simulink model "uz_pmsm_model_6LUT_pd"  (R2023b)
settings: Solver=FixedStepAuto  StartTime=0.0  StopTime=0.05  RelTol=1e-3
PreLoadFcn:
  | uz_pmsm_model_init_parameter
PostLoadFcn:
  | % Import the data from Excel for a lookup table
  | FluxMapData = readtable('C:\Users\Philipp\ultrazohm\ultrazohm_sw\ip_cores\uz_pmsm_model\FluxMapData_2023-05-26_13-07-57.csv');
  | % Row indices for lookup table
  | d_current_in_d_axis = FluxMapData(8:27,1:end);
  | % Column indices for lookup table
  | q_current_in_d_axis = FluxMapData(29:48,1:end);
  | % Output values for lookup table
  | d_Flux_d_axis = FluxMapData(50:69,1:end);
values from neighbouring files (symbols this model uses):
  ad1 = 7.2940    (= 7.294)    [LUT_approx_methode1_u_2b.m]    (also in LUT_approx_methode1_u_2b_alt.m; LUT_approx_methode2a.m = ad_1(1); LUT_approx_methode_2a_FEM.m = ad_1(1); LUT_approx_new.m = ad_1(1))
  ad2 = 0.0001    [LUT_approx_methode1_u_2b.m]    (also in LUT_approx_methode1_u_2b_alt.m; LUT_approx_methode2a.m = ad_1(2); LUT_approx_methode_2a_FEM.m = ad_1(2); LUT_approx_new.m = ad_1(2))
  ad3 = -15.5992    [LUT_approx_methode1_u_2b.m]    (also in LUT_approx_methode1_u_2b_alt.m; LUT_approx_methode2a.m = ad_1(3); LUT_approx_methode_2a_FEM.m = ad_1(3); LUT_approx_new.m = ad_1(3))
  ad4 = -186.4725    [LUT_approx_methode1_u_2b.m]    (also in LUT_approx_methode1_u_2b_alt.m; LUT_approx_methode2a.m = ad_3_6(1); LUT_approx_methode_2a_FEM.m = ad_3_6(1); LUT_approx_new.m = ad_3_6(1))
  ad5 = 187.4853    [LUT_approx_methode1_u_2b.m]    (also in LUT_approx_methode1_u_2b_alt.m; LUT_approx_methode2a.m = ad_3_6(2); LUT_approx_methode_2a_FEM.m = ad_3_6(2); LUT_approx_new.m = ad_3_6(2))
  ad6 = 0.0000    (= 0)    [LUT_approx_methode1_u_2b.m]    (also in LUT_approx_methode1_u_2b_alt.m; LUT_approx_methode2a.m = ad_3_6(3); LUT_approx_methode_2a_FEM.m = ad_3_6(3); LUT_approx_new.m = ad_3_6(3))
  aq1 = 0.0041    [LUT_approx_methode1_u_2b.m]    (also in LUT_approx_methode1_u_2b_alt.m; LUT_approx_methode2a.m = aq_1(1); LUT_approx_methode_2a_FEM.m = aq_1(1); LUT_approx_new.m = aq_1(1))
  aq2 = 0.2092    [LUT_approx_methode1_u_2b.m]    (also in LUT_approx_methode1_u_2b_alt.m; LUT_approx_methode2a.m = aq_1(2); LUT_approx_methode_2a_FEM.m = aq_1(2); LUT_approx_new.m = aq_1(2))
  aq3 = 0.0010    (= 0.001)    [LUT_approx_methode1_u_2b.m]    (also in LUT_approx_methode1_u_2b_alt.m; LUT_approx_methode2a.m = aq_1(3); LUT_approx_methode_2a_FEM.m = aq_1(3); LUT_approx_new.m = aq_1(3))
  aq4 = 28.4940    (= 28.494)    [LUT_approx_methode1_u_2b.m]    (also in LUT_approx_methode1_u_2b_alt.m; LUT_approx_methode2a.m = aq_3_6(1); LUT_approx_methode_2a_FEM.m = aq_3_6(1); LUT_approx_new.m = aq_3_6(1))
  aq5 = -24.2348    [LUT_approx_methode1_u_2b.m]    (also in LUT_approx_methode1_u_2b_alt.m; LUT_approx_methode2a.m = aq_3_6(2); LUT_approx_methode_2a_FEM.m = aq_3_6(2); LUT_approx_new.m = aq_3_6(2))
  aq6 = 0.0405    [LUT_approx_methode1_u_2b.m]    (also in LUT_approx_methode1_u_2b_alt.m; LUT_approx_methode2a.m = aq_3_6(3); LUT_approx_methode_2a_FEM.m = aq_3_6(3); LUT_approx_new.m = aq_3_6(3))
  d_current_d_Flux = FluxMapData{1,1:20}    [uz_pmsm_model_6LUT_pd_init_parameter.m]
  d_current_q_Flux = FluxMapData{66,1:20}    [uz_pmsm_model_6LUT_pd_init_parameter.m]
  entkopplung_dynamic = false    [uz_pmsm_model_6LUT_pd_init_parameter.m]
  entkopplung_linear = true    [uz_pmsm_model_6LUT_pd_init_parameter.m]
  entkopplung_static = false    [uz_pmsm_model_6LUT_pd_init_parameter.m]
  Fid1_Giq1 = ((1/2).*(aq3-aq6).*((q_current_set).^2))+((aq1./aq2).*log(cosh(aq2.*q_current_set)))-((aq4/aq5).*log(cosh(aq5.*q_current_set)))    [LUT_approx_methode2a.m]    (also in LUT_approx_methode_2a_FEM.m = (1/2).*(aq3-aq6).*((q_current_set).^2)+((aq1./aq2).*log(cosh; LUT_approx_new.m = (1/2)*(aq3-aq6)*((q_current_set).^2)+((aq1/aq2)*log(cosh(aq2; LUT_approximation_fitting.m = (1/2)*(aq3-aq6)*((iq1)^2)+((aq1/aq2)*log(cosh(aq2*iq1)))-((a)
  Fid2_Giq2 = ((ad1./ad2).*(log(cosh(ad2.*(d_current_set-ad3))))) - ((ad4./ad5).*(log(cosh(ad5.*(d_current_set-ad6)))))    [LUT_approx_methode2a.m]    (also in LUT_approx_methode_2a_FEM.m = ((ad1./ad2).*(log(cosh(ad2.*(d_current_set-ad3))))) - (((ad1)
  Flux_d = FluxMapData{43:62,1:20}'*(1e-3)    [uz_pmsm_model_6LUT_pd_init_parameter.m]
  Flux_q = FluxMapData{108:127,1:20}'*(1e-3)    [uz_pmsm_model_6LUT_pd_init_parameter.m]
  friction_coefficient = 0.001    [uz_pmsm_model_6LUT_pd_init_parameter.m]
  inertia = 0.000084    (= 8.4e-05)    [uz_pmsm_model_6LUT_pd_init_parameter.m]
  L_d = 0.00045    [uz_pmsm_model_6LUT_pd_init_parameter.m]
  L_q = 0.002    [uz_pmsm_model_6LUT_pd_init_parameter.m]
  parameter_nachfuerung = true    [uz_pmsm_model_6LUT_pd_init_parameter.m]
  polepair = 4    [uz_pmsm_model_6LUT_pd_init_parameter.m]
  praediktion_entkopplung_nonlinear = true    [uz_pmsm_model_6LUT_pd_init_parameter.m]
  psi_pm = 0.0194    [uz_pmsm_model_6LUT_pd_init_parameter.m]
  q_current_d_Flux = FluxMapData{22:41,1}    [uz_pmsm_model_6LUT_pd_init_parameter.m]
  q_current_q_Flux = FluxMapData{87:106,1}    [uz_pmsm_model_6LUT_pd_init_parameter.m]
  R_1 = 0.3    [uz_pmsm_model_6LUT_pd_init_parameter.m]
  simulate_mechanical = false    [uz_pmsm_model_6LUT_pd_init_parameter.m]
  simulate_nonlinear_modell = true    [uz_pmsm_model_6LUT_pd_init_parameter.m]
  simulate_open_loop = false    [uz_pmsm_model_6LUT_pd_init_parameter.m]
  static_friction_torque = 0.01    [uz_pmsm_model_6LUT_pd_init_parameter.m]
  tau_sum = 2*ts_regler    (= 8e-05)    [uz_pmsm_model_6LUT_pd_init_parameter.m]
  ts = 1/5e5    (= 2e-06)    [uz_pmsm_model_6LUT_pd_init_parameter.m]
  ts_regler = 1/25e3    (= 4e-05)    [uz_pmsm_model_6LUT_pd_init_parameter.m]
undefined symbols (not defined in the file or in its folder): Ki_Bo_d, Ki_Bo_q, Kp_Bo_d, Kp_Bo_q, Ldq
libraries: slpidlib x2
(part 2 of 2)

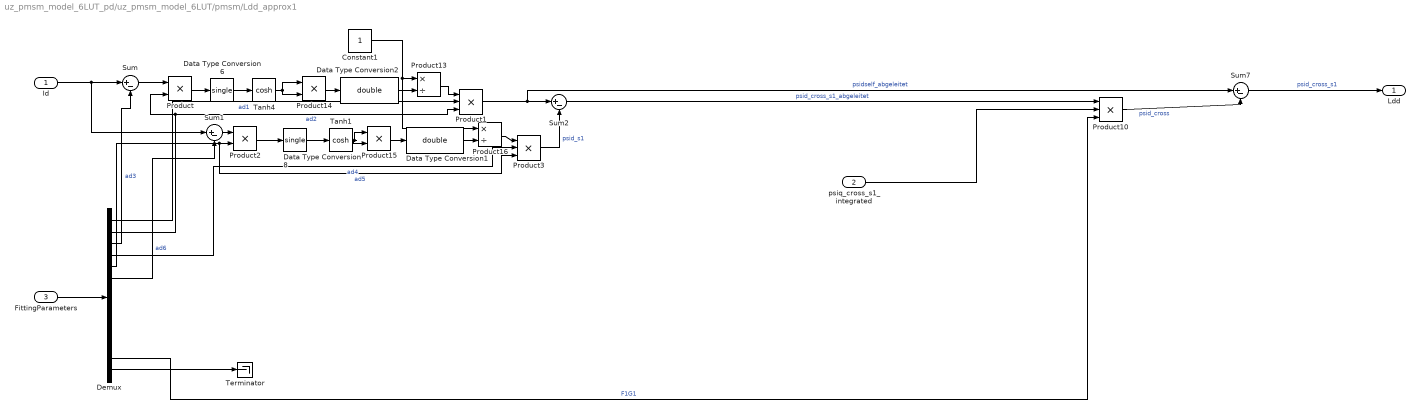
== system uz_pmsm_model_6LUT_pd/uz_pmsm_model_6LUT/pmsm/Ldd_approx1 ==
  Id : Inport
  psiq_cross_s1_integrated : Inport  Port=2
  FittingParameters : Inport  Port=3
  Constant1 : Constant  SampleTime=ts
  Data Type Conversion1 : DataTypeConversion  OutDataTypeStr=double  RndMeth=Nearest  SaturateOnIntegerOverflow=off
  Data Type Conversion2 : DataTypeConversion  OutDataTypeStr=double  RndMeth=Nearest  SaturateOnIntegerOverflow=off
  Data Type Conversion6 : DataTypeConversion  OutDataTypeStr=single  RndMeth=Nearest  SaturateOnIntegerOverflow=off
  Data Type Conversion8 : DataTypeConversion  OutDataTypeStr=single  RndMeth=Nearest  SaturateOnIntegerOverflow=off
  Demux : Demux  Outputs=14
  Product : Product
  Product1 : Product  Inputs=3
  Product10 : Product  Inputs=3
  Product13 : Product  Inputs=*/
  Product14 : Product
  Product15 : Product
  Product16 : Product  Inputs=*/
  Product2 : Product  OutDataTypeStr=Inherit: Same as first input
  Product3 : Product  Inputs=3
  Sum{,1..2,7} (4 alike) : Sum  Inputs=|+-
  Tanh1 : Trigonometry  Operator=cosh
  Tanh4 : Trigonometry  Operator=cosh
  Terminator : Terminator
  Ldd : Outport
  wires:
  FittingParameters/1 -> Demux/1
  Demux/1 -> Product1/2  "ad1"
  Demux/3 -> Sum/2  "ad3"
  Sum/1 -> Product/1
  Demux/2 -> Product1/3, Product/2  "ad2"
  Product/1 -> Data Type Conversion6/1
  Product13/1 -> Product1/1
  Product1/1 -> Sum7/1, Sum2/1  "psidself_abgeleitet"
  Demux/4 -> Product3/2  "ad4"
  Sum1/1 -> Product2/1
  Demux/5 -> Product3/3, Product2/2  "ad5"
  Demux/6 -> Sum1/2  "ad6"
  Id/1 -> Sum1/1, Sum/1
  Product3/1 -> Sum2/2  "psid_s1"
  Product2/1 -> Data Type Conversion8/1
  Sum2/1 -> Product10/1  "psid_cross_s1_abgeleitet"
  Product10/1 -> Sum7/2  "psid_cross"
  Sum7/1 -> Ldd/1  "psid_cross_s1"
  Demux/14 -> Terminator/1
  Demux/13 -> Product10/3  "F1G1"
  Product14/1 -> Data Type Conversion2/1
  Tanh4/1 -> Product14/1, Product14/2
  Constant1/1 -> Product16/1, Product13/1
  Tanh1/1 -> Product15/2, Product15/1
  Product16/1 -> Product3/1
  Product15/1 -> Data Type Conversion1/1
  Data Type Conversion1/1 -> Product16/2
  Data Type Conversion2/1 -> Product13/2
  Data Type Conversion6/1 -> Tanh4/1
  Data Type Conversion8/1 -> Tanh1/1
  psiq_cross_s1_integrated/1 -> Product10/2

== system uz_pmsm_model_6LUT_pd/uz_pmsm_model_6LUT/pmsm/Ldq ==
  psid_cross_s1 : Inport
  psiq_cross_s1 : Inport  Port=2
  FittingParameters : Inport  Port=3
  Demux : Demux  Outputs=14
  Gain : Gain  Gain=-1
  Product20 : Product  Inputs=3
  Terminator : Terminator
  psiq : Outport
  wires:
  FittingParameters/1 -> Demux/1
  Product20/1 -> Gain/1  "psiq_cross"
  psid_cross_s1/1 -> Product20/1
  Gain/1 -> psiq/1
  Demux/14 -> Terminator/1
  Demux/13 -> Product20/3
  psiq_cross_s1/1 -> Product20/2

== system uz_pmsm_model_6LUT_pd/uz_pmsm_model_6LUT/pmsm/Lqd ==
  psid_cross_s1 : Inport
  psiq_cross_s1 : Inport  Port=2
  FittingParameters : Inport  Port=3
  Demux : Demux  Outputs=14
  Gain : Gain  Gain=-1
  Product20 : Product  Inputs=3
  Terminator : Terminator
  psiq : Outport
  wires:
  FittingParameters/1 -> Demux/1
  Product20/1 -> Gain/1  "psiq_cross"
  Demux/13 -> Terminator/1
  psid_cross_s1/1 -> Product20/1
  Demux/14 -> Product20/3
  Gain/1 -> psiq/1
  psiq_cross_s1/1 -> Product20/2

== system uz_pmsm_model_6LUT_pd/uz_pmsm_model_6LUT/pmsm/Lqq_approx1 ==
  psid_cross_s1_integrated : Inport
  Iq : Inport  Port=2
  FittingParameters : Inport  Port=3
  Constant1 : Constant  SampleTime=ts
  Data Type Conversion2 : DataTypeConversion  OutDataTypeStr=double  RndMeth=Nearest  SaturateOnIntegerOverflow=off
  Data Type Conversion4 : DataTypeConversion  OutDataTypeStr=single  RndMeth=Nearest  SaturateOnIntegerOverflow=off
  Data Type Conversion5 : DataTypeConversion  OutDataTypeStr=single  RndMeth=Nearest  SaturateOnIntegerOverflow=off
  Data Type Conversion6 : DataTypeConversion  OutDataTypeStr=double  RndMeth=Nearest  SaturateOnIntegerOverflow=off
  Demux : Demux  Outputs=14
  Product : Product  OutDataTypeStr=Inherit: Same as first input
  Product1 : Product  Inputs=3
  Product13 : Product  Inputs=*/
  Product14 : Product
  Product15 : Product
  Product16 : Product  Inputs=*/
  Product2 : Product  OutDataTypeStr=Inherit: Same as first input
  Product20 : Product  Inputs=3
  Product3 : Product  Inputs=3
  Sum1 : Sum  Inputs=|++
  Sum10 : Sum  Inputs=|+-
  Sum2 : Sum  Inputs=|+-
  Sum4 : Sum  Inputs=|++
  Tanh1 : Trigonometry  Operator=cosh
  Tanh3 : Trigonometry  Operator=cosh
  Terminator : Terminator
  Lqq : Outport
  wires:
  FittingParameters/1 -> Demux/1
  Demux/12 -> Sum4/2  "aq6"
  Product20/1 -> Sum10/2  "psiq_cross"
  Sum10/1 -> Lqq/1  "Lqq"
  Demux/14 -> Product20/3
  Demux/13 -> Terminator/1
  Product15/1 -> Data Type Conversion2/1
  Demux/9 -> Sum1/2  "aq3"
  Constant1/1 -> Product16/1, Product13/1
  Tanh3/1 -> Product14/1, Product14/2
  Tanh1/1 -> Product15/2, Product15/1
  Sum2/1 -> Product20/1
  Product13/1 -> Product1/1
  Product16/1 -> Product3/1
  Product14/1 -> Data Type Conversion6/1
  Demux/10 -> Product3/2  "aq4"
  Demux/8 -> Product/2, Product1/3  "aq2"
  Product2/1 -> Data Type Conversion4/1
  Iq/1 -> Product2/1, Product/1
  Product/1 -> Data Type Conversion5/1
  Demux/11 -> Product2/2, Product3/3  "aq5"
  Demux/7 -> Product1/2  "aq1"
  Product1/1 -> Sum1/1  "psidself_abgeleitet"
  Sum1/1 -> Sum10/1, Sum2/1
  Sum4/1 -> Sum2/2
  Product3/1 -> Sum4/1  "psid_s1"
  Data Type Conversion2/1 -> Product16/2
  Data Type Conversion4/1 -> Tanh1/1
  Data Type Conversion5/1 -> Tanh3/1
  Data Type Conversion6/1 -> Product13/2
  psid_cross_s1_integrated/1 -> Product20/2

== system uz_pmsm_model_6LUT_pd/uz_pmsm_model_6LUT/pmsm/Subsystem ==
  in : Inport
  reset : Inport  Port=2
  Delay1 : Delay  DelayLength=1  ExternalReset=Level
      settings: InputPortMap=u0,r5
  Gain7 : Gain  Gain=ts
  Sum5 : Sum  Inputs=|++
  outt : Outport
  wires:
  in/1 -> Gain7/1
  reset/1 -> Delay1/2
  Delay1/1 -> outt/1, Sum5/2
  Sum5/1 -> Delay1/1
  Gain7/1 -> Sum5/1  "u_d"

== system uz_pmsm_model_6LUT_pd/uz_pmsm_model_6LUT/pmsm/Subsystem1 ==
  in : Inport
  reset : Inport  Port=2
  Delay1 : Delay  DelayLength=1  ExternalReset=Level
      settings: InputPortMap=u0,r5
  Gain7 : Gain  Gain=ts
  Sum5 : Sum  Inputs=|++
  outt : Outport
  wires:
  in/1 -> Gain7/1
  reset/1 -> Delay1/2
  Delay1/1 -> outt/1, Sum5/2
  Sum5/1 -> Delay1/1
  Gain7/1 -> Sum5/1  "u_d"

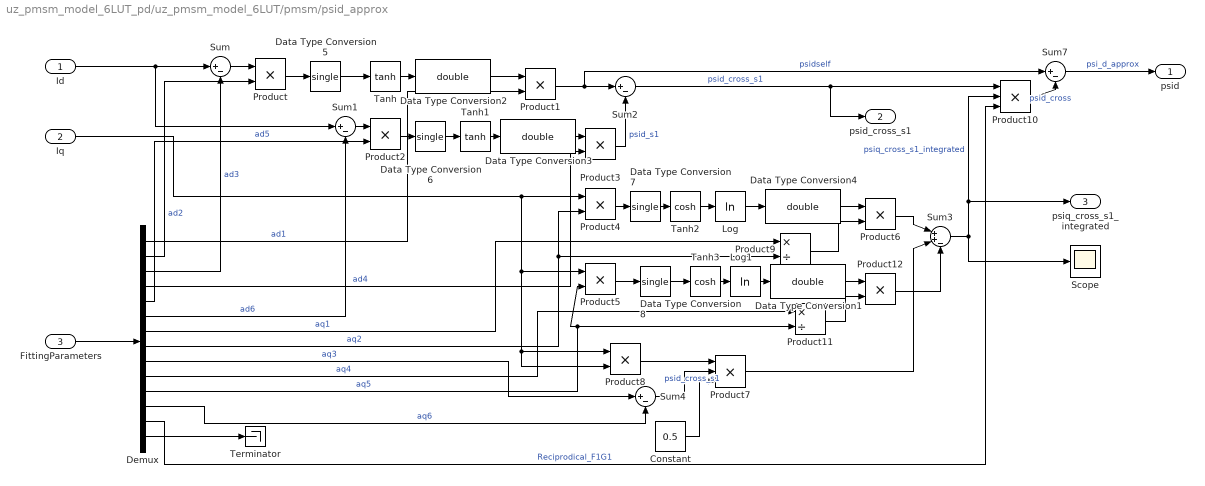
== system uz_pmsm_model_6LUT_pd/uz_pmsm_model_6LUT/pmsm/psid_approx ==
  Id : Inport
  Iq : Inport  Port=2
  FittingParameters : Inport  Port=3
  Constant : Constant  Value=0.5  SampleTime=-1
  Data Type Conversion{1..4} (4 alike) : DataTypeConversion  OutDataTypeStr=double  RndMeth=Nearest  SaturateOnIntegerOverflow=off
  Data Type Conversion{5..8} (4 alike) : DataTypeConversion  OutDataTypeStr=single  RndMeth=Nearest  SaturateOnIntegerOverflow=off
  Demux : Demux  Outputs=14
  Log : Math  Operator=log  SignedPower=on
  Log1 : Math  Operator=log  SignedPower=on
  Product{,2,4..5} (4 alike) : Product  OutDataTypeStr=Inherit: Same as first input
  Product{1,3,6,8,12} (5 alike) : Product
  Product10 : Product  Inputs=3
  Product11 : Product  Inputs=*/
  Product7 : Product  Inputs=3
  Product9 : Product  Inputs=*/
  Scope : Scope
  Sum{,1..2,4,7} (5 alike) : Sum  Inputs=|+-
  Sum3 : Sum  Inputs=|++-
  Tanh : Trigonometry  Operator=tanh
  Tanh1 : Trigonometry  Operator=tanh
  Tanh2 : Trigonometry  Operator=cosh
  Tanh3 : Trigonometry  Operator=cosh
  Terminator : Terminator
  psid : Outport
  psid_cross_s1 : Outport  Port=2
  psiq_cross_s1_integrated : Outport  Port=3
  wires:
  FittingParameters/1 -> Demux/1
  Demux/1 -> Product1/2  "ad1"
  Demux/3 -> Sum/2  "ad3"
  Sum/1 -> Product/1
  Demux/2 -> Product/2  "ad2"
  Product/1 -> Data Type Conversion5/1
  Tanh/1 -> Data Type Conversion2/1
  Product1/1 -> Sum7/1, Sum2/1  "psidself"
  Demux/4 -> Product3/2  "ad4"
  Sum1/1 -> Product2/1
  Demux/5 -> Product2/2  "ad5"
  Demux/6 -> Sum1/2  "ad6"
  Tanh1/1 -> Data Type Conversion3/1
  Id/1 -> Sum1/1, Sum/1
  Product3/1 -> Sum2/2  "psid_s1"
  Iq/1 -> Product8/2, Product8/1, Product5/1, Product4/1
  Sum2/1 -> psid_cross_s1/1, Product10/1  "psid_cross_s1"
  Tanh2/1 -> Log/1
  Tanh3/1 -> Log1/1
  Product5/1 -> Data Type Conversion8/1
  Sum4/1 -> Product7/2  "psid_cross_s1"
  Product8/1 -> Product7/1
  Product7/1 -> Sum3/2
  Product9/1 -> Product6/2
  Log/1 -> Data Type Conversion4/1
  Product6/1 -> Sum3/1
  Product11/1 -> Product12/2
  Log1/1 -> Data Type Conversion1/1
  Product12/1 -> Sum3/3
  Constant/1 -> Product7/3
  Sum3/1 -> Product10/2, psiq_cross_s1_integrated/1, Scope/1  "psiq_cross_s1_integrated"
  Demux/10 -> Product11/1  "aq4"
  Demux/7 -> Product9/1  "aq1"
  Demux/9 -> Sum4/1  "aq3"
  Demux/11 -> Product5/2, Product11/2  "aq5"
  Demux/8 -> Product4/2, Product9/2  "aq2"
  Demux/12 -> Sum4/2  "aq6"
  Product10/1 -> Sum7/2  "psid_cross"
  Sum7/1 -> psid/1  "psi_d_approx"
  Demux/14 -> Terminator/1
  Demux/13 -> Product10/3  "Reciprodical_F1G1"
  Data Type Conversion4/1 -> Product6/1
  Data Type Conversion1/1 -> Product12/1
  Data Type Conversion2/1 -> Product1/1
  Data Type Conversion3/1 -> Product3/1
  Data Type Conversion5/1 -> Tanh/1
  Product2/1 -> Data Type Conversion6/1
  Data Type Conversion6/1 -> Tanh1/1
  Data Type Conversion7/1 -> Tanh2/1
  Product4/1 -> Data Type Conversion7/1
  Data Type Conversion8/1 -> Tanh3/1

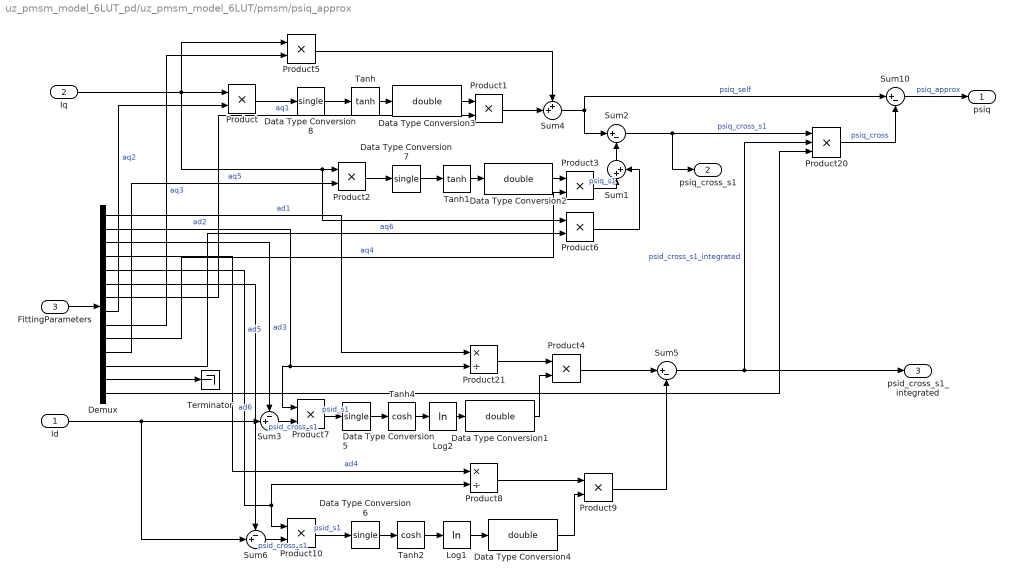
== system uz_pmsm_model_6LUT_pd/uz_pmsm_model_6LUT/pmsm/psiq_approx ==
  Id : Inport
  Iq : Inport  Port=2
  FittingParameters : Inport  Port=3
  Data Type Conversion{1..4} (4 alike) : DataTypeConversion  OutDataTypeStr=double  RndMeth=Nearest  SaturateOnIntegerOverflow=off
  Data Type Conversion{5..8} (4 alike) : DataTypeConversion  OutDataTypeStr=single  RndMeth=Nearest  SaturateOnIntegerOverflow=off
  Demux : Demux  Outputs=14
  Log1 : Math  Operator=log  SignedPower=on
  Log2 : Math  Operator=log  SignedPower=on
  Product{,2,7,10} (4 alike) : Product  OutDataTypeStr=Inherit: Same as first input
  Product{1,3..6,9} (6 alike) : Product
  Product20 : Product  Inputs=3
  Product21 : Product  Inputs=*/
  Product8 : Product  Inputs=*/
  Sum1 : Sum  Inputs=|++
  Sum10 : Sum  Inputs=|+-
  Sum2 : Sum  Inputs=|+-
  Sum3 : Sum  Inputs=-+|
  Sum4 : Sum  Inputs=++|
  Sum5 : Sum  Inputs=|+-
  Sum6 : Sum  Inputs=-+|
  Tanh : Trigonometry  Operator=tanh
  Tanh1 : Trigonometry  Operator=tanh
  Tanh2 : Trigonometry  Operator=cosh
  Tanh4 : Trigonometry  Operator=cosh
  Terminator : Terminator
  psiq : Outport
  psiq_cross_s1 : Outport  Port=2
  psid_cross_s1_integrated : Outport  Port=3
  wires:
  FittingParameters/1 -> Demux/1
  Sum2/1 -> Product20/1, psiq_cross_s1/1  "psiq_cross_s1"
  Demux/10 -> Product3/2  "aq4"
  Product2/1 -> Data Type Conversion7/1
  Demux/12 -> Product6/2  "aq6"
  Demux/8 -> Product/2  "aq2"
  Product/1 -> Data Type Conversion8/1
  Demux/11 -> Product2/2  "aq5"
  Tanh/1 -> Data Type Conversion3/1
  Demux/7 -> Product1/2  "aq1"
  Tanh1/1 -> Data Type Conversion2/1
  Iq/1 -> Product2/1, Product6/1, Product/1, Product5/1
  Demux/9 -> Product5/2  "aq3"
  Log2/1 -> Data Type Conversion1/1
  Tanh4/1 -> Log2/1
  Product21/1 -> Product4/1
  Product1/1 -> Sum4/2
  Product5/1 -> Sum4/1
  Sum4/1 -> Sum10/1, Sum2/1  "psiq_self"
  Sum1/1 -> Sum2/2
  Product3/1 -> Sum1/1  "psiq_s1"
  Product6/1 -> Sum1/2
  Sum3/1 -> Product7/2  "psid_cross_s1"
  Product7/1 -> Data Type Conversion5/1  "psid_s1"
  Product4/1 -> Sum5/1
  Product9/1 -> Sum5/2
  Product10/1 -> Data Type Conversion6/1  "psid_s1"
  Tanh2/1 -> Log1/1
  Product8/1 -> Product9/1
  Log1/1 -> Data Type Conversion4/1
  Sum6/1 -> Product10/2  "psid_cross_s1"
  Demux/3 -> Sum3/1  "ad3"
  Demux/1 -> Product21/1  "ad1"
  Demux/4 -> Product8/1  "ad4"
  Demux/2 -> Product7/1, Product21/2  "ad2"
  Demux/5 -> Product8/2, Product10/1  "ad5"
  Demux/6 -> Sum6/1  "ad6"
  Id/1 -> Sum6/2, Sum3/2
  Sum5/1 -> Product20/2, psid_cross_s1_integrated/1  "psid_cross_s1_integrated"
  Product20/1 -> Sum10/2  "psiq_cross"
  Sum10/1 -> psiq/1  "psiq_approx"
  Demux/14 -> Product20/3
  Demux/13 -> Terminator/1
  Data Type Conversion4/1 -> Product9/2
  Data Type Conversion1/1 -> Product4/2
  Data Type Conversion2/1 -> Product3/1
  Data Type Conversion3/1 -> Product1/1
  Data Type Conversion5/1 -> Tanh4/1
  Data Type Conversion6/1 -> Tanh2/1
  Data Type Conversion7/1 -> Tanh1/1
  Data Type Conversion8/1 -> Tanh/1
